simulink model "spiBitbangSimulink_So2"  (R2013b)
settings: Solver=FixedStepDiscrete  SolverMode=SingleTasking  StartTime=0.0  StopTime=4e-3  FixedStep=sampleTime  MaxStep=MaxStepSize  RelTol=1e-3
undefined symbols (not defined in the file or in its folder): Low, periSam, sampleTime, sampleTIme, sigbuilder_block
libraries: simulink_extras x30, simulink x16, dspswit3 x8, embdlinuxlib x5, powerlib_meascontrol x2, dspsnks4 x1
settings Model: ExtModeTrigDuration=100  Creator=mainster  LastModifiedBy=mainster
settings OptimizationCC: OptimizeModelRefInitCode=on  LifeSpan=1
settings DebuggingCC: SolverPrmCheckMsg=none  InheritedTsInSrcMsg=none
settings HardwareCC: ProdLargestAtomicInteger=Long  ProdLargestAtomicFloat=Double  ProdEndianess=LittleEndian  ProdHWDeviceType=ARM Compatible->ARM Cortex
settings RTWCC: SystemTargetFile=realtime.tlc  GenerateMakefile=off  TemplateMakefile=realtime.tmf  Description=Run on Target Hardware  RTWVerbose=off  ProcessScript=realtime_make_rtw_hook
settings STFCustomTargetCC: TargetLibSuffix=.a  GenerateSampleERTMain=on  ERTCustomFileBanners=on  SupportNonInlinedSFcns=off  SupportVariableSizeSignals=on  MATLABClassNameForMDSCustomization=Simulink.SoftwareTarget.ERTCustomization  GRTInterface=off  SystemTargetFile=realtime.tlc
settings ERTTargetCC: CodeReplacementLibrary=ANSI_C  GenerateSampleERTMain=on  ParMdlRefBuildCompliant=off  CompOptLevelCompliant=off  ConcurrentExecutionCompliant=off  CombineOutputUpdateFcns=off  ERTFirstTimeCompliant=off  SupportContinuousTime=on  SupportVariableSizeSignals=on  ModelStepFunctionPrototypeControlCompliant=off  CPPClassGenCompliant=off  ExtModeMexArgs='192.168.2.111' 0 17725  InlinedParameterPlacement=NonHierarchical  ERTSrcFileBannerTemplate=realtime_code_template.cgt  ERTHdrFileBannerTemplate=realtime_code_template.cgt  ERTDataSrcFileTemplate=realtime_code_template.cgt  ERTDataHdrFileTemplate=realtime_code_template.cgt  ERTCustomFileTemplate=realtime_file_process.tlc
settings ConfigurationSet: Description=SimMechanics 2G

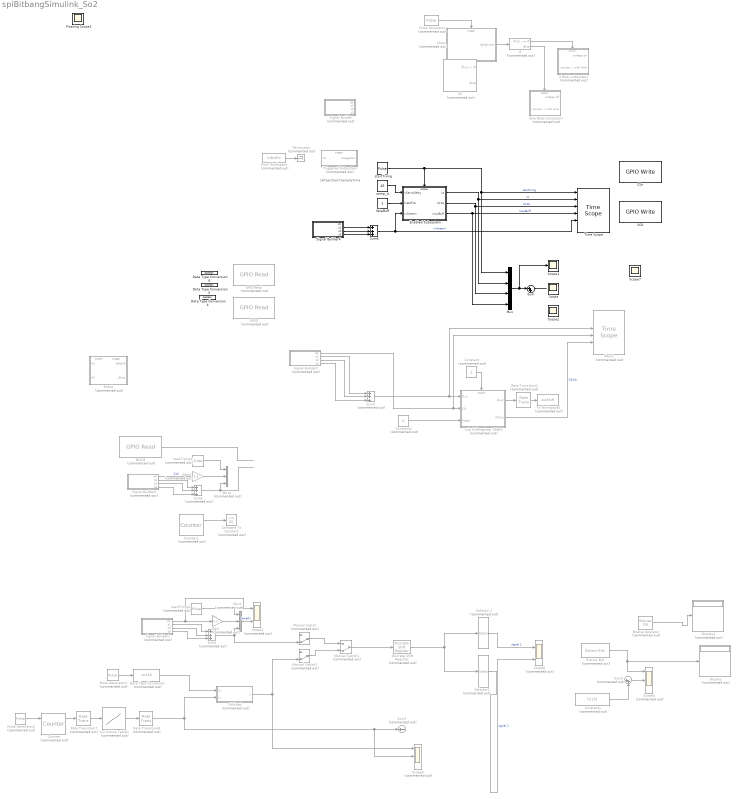
== system spiBitbangSimulink_So2 ==
  note: 16*periSam*sampleTime
  " ShiftLeft" : Subsystem  Commented=on  TreatAsAtomicUnit=on
  1-D Lookup Table1 : Lookup_n-D  Commented=on  NumberOfTableDimensions=1  BreakpointsForDimension1=[0,1,2,3,4]  IndexSearchMethod=Evenly spaced points  UseOneInputPortForAllInputData=on  Table=[3325,6553,44558,8856,60254]  TableDataTypeStr=uint16  InterpMethod=Flat  SampleTime=sampleTime  InternalRulePriority=Speed  OutDataTypeStr=uint16  RndMeth=Simplest  InputSameDT=on
  Bitwise Operator : simulink/Logic and Bit Operations/Bitwise Operator  Commented=on  logicop=OR  UseBitMask=off  BitMask=bin2dec('11011001')  BitMaskRealWorld=Real World Value
  CSn : embdlinuxlib/GPIO Write  board=Model B Rev2  gpio=27  direction=Output  blockPlatform=Raspberry Pi
  Chart : Stateflow chart  Commented=on  TreatAsAtomicUnit=on
  Compare To Constant : simulink/Logic and Bit Operations/Compare To Constant  Commented=on  relop=<=  const=25  OutDataTypeStr=boolean  ZeroCross=off
  Constant : Constant  Commented=on  SampleTime=-1
  Constant1 : Constant  Commented=on  Value=[0:15]  VectorParams1D=off  SampleTime=sampleTIme
      settings: SamplingMode=Frame based
  Constant2 : Constant  Commented=on  Value=0  OutDataTypeStr=Inherit: Inherit via back propagation  SampleTime=-1
  Counter : dspswit3/Counter  Commented=on  Direction=Up  CountEvent=Rising edge  CounterSize=User defined  MaxCount=5  InitialCount=1  Output=Count and Hit  HitValue=32  ResetInput=on  SamplesPerFrame=1  Ts=1  CntDtype=double  HitDtype=Logical
  Counter1 : dspswit3/Counter  Commented=on  Direction=Up  CountEvent=Rising edge  CounterSize=User defined  MaxCount=255  InitialCount=0  Output=Count and Hit  HitValue=32  ResetInput=on  SamplesPerFrame=1  Ts=1  CntDtype=double  HitDtype=Boolean
  Data Type Conversion : DataTypeConversion  Commented=on  OutDataTypeStr=uint16
  Data Type Conversion4 : DataTypeConversion  OutDataTypeStr=boolean
  Data Type Conversion5 : DataTypeConversion  OutDataTypeStr=boolean
  Data Type Conversion6 : DataTypeConversion  OutDataTypeStr=boolean
  Discrete Shift Register : powerlib_meascontrol/Additional Components/Discrete Shift Register  Commented=on  NSamples=16  InitialValue=0  Ts=periSam*sampleTime
  Display : Display  Commented=on
      settings: Format=decimal (Stored Integer)
  Display1 : Display  Commented=on
      settings: Format=decimal (Stored Integer)
  Else Body subsystem : Subsystem  Commented=on  TreatAsAtomicUnit=on
  Enabled Subsystem : Subsystem  TreatAsAtomicUnit=on
  Extract Bits : simulink/Logic and Bit Operations/Extract Bits  Commented=on  bitsToExtract=Range of bits  numBits=8  bitIdxRange=[0 0]  outScalingMode=Treat bit field as an integer
  From Workspace : FromWorkspace  Commented=on  VariableName=txBuffIn  SampleTime=0
  GPIO Read : embdlinuxlib/GPIO Read  Commented=on  board=Model B Rev2  gpio=4  internalResistor=Off  sampleTime=0.1  direction=Input  blockPlatform=Raspberry Pi
  Gain : Gain  Commented=on  Gain=1.1  SampleTime=sampleTime
  Gain2 : Gain  Commented=on  Gain=1.1  SampleTime=sampleTime
  If : If  Commented=on  IfExpression=u1 ~= 0
  If Body subsystem : Subsystem  Commented=on  TreatAsAtomicUnit=on
  If1 : If  Commented=on  NumInputs=2
  MISO : embdlinuxlib/GPIO Read  Commented=on  board=Model B Rev2  gpio=24  internalResistor=Off  sampleTime=0.1  direction=Input  blockPlatform=Raspberry Pi
  MISO1 : embdlinuxlib/GPIO Read  Commented=on  board=Model B Rev2  gpio=4  internalResistor=Off  sampleTime=0.1  direction=Input  blockPlatform=Raspberry Pi
  Main1 : TimeScope  Commented=on  NumInputPorts=6  DefaultConfigurationName=spbscopes.TimeScopeBlockCfg
      settings: CopyFcn=scopeextensions.ScopeBlock.onCoreBlockCopy(gcbh);  DeleteFcn=scopeextensions.ScopeBlock.callback(gcbh, 'onBlockDelete');  PreSaveFcn=scopeextensions.ScopeBlock.callback(gcbh, 'onModelSave');  NameChangeFcn=scopeextensions.ScopeBlock.callback(gcbh, 'onBlockRename');  DestroyFcn=scopeextensions.ScopeBlock.onBlockDestroy(gcbh)  CloseFcn=scopeextensions.ScopeBlock.callback(gcbh, 'onBlockClose');  PreDeleteFcn=scopeextensions.ScopeBlock.callback(gcbh, 'onBlockPreDelete');
  Manual Switch : ManualSwitch  Commented=on  CurrentSetting=0
  Manual Switch1 : ManualSwitch  Commented=on  CurrentSetting=0
  Manual Switch2 : ManualSwitch  Commented=on  CurrentSetting=0
  Mux : Mux
  Mux1 : Mux  Commented=on  Inputs=3
  Mux4 : Mux  Commented=on  Inputs=3
  Pulse Generator : DiscretePulseGenerator  Commented=on  Period=periSam  PulseWidth=periSam/2  SampleTime=-1
  Pulse Generator1 : DiscretePulseGenerator  Commented=on  Period=periSam  PulseWidth=periSam/2  SampleTime=periSam*sampleTime
  Pulse Generator2 : DiscretePulseGenerator  Commented=on  Period=periSam*16  PulseWidth=8*periSam  SampleTime=sampleTime
  Rate Transition1 : RateTransition  Commented=on  OutPortSampleTime=sampleTime*periSam
  Rate Transition7 : RateTransition  Commented=on  OutPortSampleTime=sampleTime
  Rate Transition8 : RateTransition  Commented=on  OutPortSampleTime=periSam*sampleTime
  RxSub : Subsystem  Commented=on  TreatAsAtomicUnit=on
  SCK : embdlinuxlib/GPIO Write  board=Model B Rev2  gpio=17  direction=Output  blockPlatform=Raspberry Pi
  Scope : Scope
      settings: Floating=on  ShowLegends=on  TimeRange=0.002  YMin=-0.2
  Scope1 : Scope
      settings: ShowLegends=on  TimeRange=0.002  YMin=-0.2
  Scope2 : Scope  NumInputPorts=4
      settings: Floating=on  ShowLegends=on  TimeRange=0.002  YMin=-0.2~-0.2~-0.2~-0.2  YMax=1.2~1.2~1.2~18  SaveName=ScopeData2
  Scope3 : Scope  Commented=on  NumInputPorts=2
      settings: ShowLegends=on  TimeRange=0.00032  YMin=-0.2~-5  YMax=1.6~5  SaveName=ScopeData4  SampleInput=on
  Scope4 : Scope  Commented=on  NumInputPorts=3
      settings: ShowLegends=on  TimeRange=0.00032  YMin=-0.2~-5~-5  YMax=1.6~5~5  SaveName=ScopeData5  SampleInput=on
  Scope5 : Scope  Commented=on  NumInputPorts=3
      settings: ShowLegends=on  TimeRange=0.00032  YMin=-0.2~-5~-5  YMax=1.6~5~5  SaveName=ScopeData6  SampleInput=on
  Scope6 : Scope  Commented=on  NumInputPorts=2
      settings: TimeRange=0.03  YMin=-1~-1  YMax=1~1  SaveName=ScopeData7
  Scope7 : Scope  NumInputPorts=4
      settings: ShowLegends=on  TimeRange=0.004  YMin=-0.2~-0.2~-0.2~-0.2  YMax=1.2~1.2~1.2~18  SaveName=ScopeData9
  Selector 1 : Selector  Commented=on  InputPortWidth=16  IndexOptions=Index vector (dialog)  Indices=[1:8]  OutputSizes=1
  Selector2 : Selector  Commented=on  InputPortWidth=16  IndexOptions=Index vector (dialog)  Indices=[9:16]  OutputSizes=1
  Signal Builder : Subsystem  Tag=STV Subsys  Commented=on  LoadFcn=sigbuilder_block('load');  StartFcn=sigbuilder_block('start');  StopFcn=sigbuilder_block('stop');  ClipboardFcn=sigbuilder_block('clipboard');  mask(Sigbuilder block){}
      mask help: Simulink:masks:SigbuilderBlock_MD
      mask init:
      | if ~strcmp(get_param(bdroot(gcbh),'SimulationStatus'),'stopped') tuvar = sigbuilder_block('maskInit'); end
      settings: CopyFcn=sigbuilder_block('copy');  DeleteFcn=sigbuilder_block('delete');  ModelCloseFcn=sigbuilder_block('modelClose');  PreSaveFcn=sigbuilder_block('preSave');  PauseFcn=sigbuilder_block('pause');  ContinueFcn=sigbuilder_block('continue');  NameChangeFcn=sigbuilder_block('namechange');  OpenFcn=sigbuilder_block('open',[141 95.25 837.75 399.75 ]);  CloseFcn=sigbuilder_block('close');
      mask Display: plot(0, 0, 100, 100,[2, 2, 32, 32, 2], [68, 8, 8, 68, 68],[32, 2], [38, 38], [32, 19, 2],[53, 60, 44], [32, 17, 17, 2],[16, 16, 31, 31]);txt = getActiveGroup(gcbh);text(2, 100, txt,'verticalAlignment', 'top');
  Signal Builder1 : Subsystem  Tag=STV Subsys  Commented=on  LoadFcn=sigbuilder_block('load');  StartFcn=sigbuilder_block('start');  StopFcn=sigbuilder_block('stop');  ClipboardFcn=sigbuilder_block('clipboard');  mask(Sigbuilder block){}
      mask help: Simulink:masks:SigbuilderBlock_MD
      mask init:
      | if ~strcmp(get_param(bdroot(gcbh),'SimulationStatus'),'stopped') tuvar = sigbuilder_block('maskInit'); end
      settings: CopyFcn=sigbuilder_block('copy');  DeleteFcn=sigbuilder_block('delete');  ModelCloseFcn=sigbuilder_block('modelClose');  PreSaveFcn=sigbuilder_block('preSave');  PauseFcn=sigbuilder_block('pause');  ContinueFcn=sigbuilder_block('continue');  NameChangeFcn=sigbuilder_block('namechange');  OpenFcn=sigbuilder_block('open',[367.5 138 550.5 399.75 ]);  CloseFcn=sigbuilder_block('close');
      mask Display: plot(0, 0, 100, 100,[2, 2, 32, 32, 2], [68, 8, 8, 68, 68],[32, 2], [38, 38], [32, 19, 2],[53, 60, 44], [32, 17, 17, 2],[16, 16, 31, 31]);txt = getActiveGroup(gcbh);text(2, 100, txt,'verticalAlignment', 'top');
  Signal Builder2 : Subsystem  Tag=STV Subsys  Commented=on  LoadFcn=sigbuilder_block('load');  StartFcn=sigbuilder_block('start');  StopFcn=sigbuilder_block('stop');  ClipboardFcn=sigbuilder_block('clipboard');  TreatAsAtomicUnit=on  mask(Sigbuilder block){}
      mask help: Simulink:masks:SigbuilderBlock_MD
      mask init:
      | if ~strcmp(get_param(bdroot(gcbh),'SimulationStatus'),'stopped') tuvar = sigbuilder_block('maskInit'); end
      settings: CopyFcn=sigbuilder_block('copy');  DeleteFcn=sigbuilder_block('delete');  ModelCloseFcn=sigbuilder_block('modelClose');  PreSaveFcn=sigbuilder_block('preSave');  PauseFcn=sigbuilder_block('pause');  ContinueFcn=sigbuilder_block('continue');  NameChangeFcn=sigbuilder_block('namechange');  OpenFcn=sigbuilder_block('open',[367.5 138 550.5 399.75 ]);  CloseFcn=sigbuilder_block('close');
      mask Display: plot(0, 0, 100, 100,[2, 2, 32, 32, 2], [68, 8, 8, 68, 68],[32, 2], [38, 38], [32, 19, 2],[53, 60, 44], [32, 17, 17, 2],[16, 16, 31, 31]);txt = getActiveGroup(gcbh);text(2, 100, txt,'verticalAlignment', 'top');
  Signal Builder3 : Subsystem  Tag=STV Subsys  Commented=on  LoadFcn=sigbuilder_block('load');  StartFcn=sigbuilder_block('start');  StopFcn=sigbuilder_block('stop');  ClipboardFcn=sigbuilder_block('clipboard');  SystemSampleTime=sampleTime  mask(Sigbuilder block){}
      mask help: Simulink:masks:SigbuilderBlock_MD
      mask init:
      | if ~strcmp(get_param(bdroot(gcbh),'SimulationStatus'),'stopped') tuvar = sigbuilder_block('maskInit'); end
      settings: CopyFcn=sigbuilder_block('copy');  DeleteFcn=sigbuilder_block('delete');  ModelCloseFcn=sigbuilder_block('modelClose');  PreSaveFcn=sigbuilder_block('preSave');  PauseFcn=sigbuilder_block('pause');  ContinueFcn=sigbuilder_block('continue');  NameChangeFcn=sigbuilder_block('namechange');  OpenFcn=sigbuilder_block('open',[367.5 138 550.5 399.75 ]);  CloseFcn=sigbuilder_block('close');
      mask Display: plot(0, 0, 100, 100,[2, 2, 32, 32, 2], [68, 8, 8, 68, 68],[32, 2], [38, 38], [32, 19, 2],[53, 60, 44], [32, 17, 17, 2],[16, 16, 31, 31]);txt = getActiveGroup(gcbh);text(2, 100, txt,'verticalAlignment', 'top');
  Signal Builder4 : Subsystem  Tag=STV Subsys  LoadFcn=sigbuilder_block('load');  StartFcn=sigbuilder_block('start');  StopFcn=sigbuilder_block('stop');  ClipboardFcn=sigbuilder_block('clipboard');  TreatAsAtomicUnit=on  mask(Sigbuilder block){}
      mask help: Simulink:masks:SigbuilderBlock_MD
      mask init:
      | if ~strcmp(get_param(bdroot(gcbh),'SimulationStatus'),'stopped') tuvar = sigbuilder_block('maskInit'); end
      settings: CopyFcn=sigbuilder_block('copy');  DeleteFcn=sigbuilder_block('delete');  ModelCloseFcn=sigbuilder_block('modelClose');  PreSaveFcn=sigbuilder_block('preSave');  PauseFcn=sigbuilder_block('pause');  ContinueFcn=sigbuilder_block('continue');  NameChangeFcn=sigbuilder_block('namechange');  OpenFcn=sigbuilder_block('open',[367.5 138 550.5 399.75 ]);  CloseFcn=sigbuilder_block('close');
      mask Display: plot(0, 0, 100, 100,[2, 2, 32, 32, 2], [68, 8, 8, 68, 68],[32, 2], [38, 38], [32, 19, 2],[53, 60, 44], [32, 17, 17, 2],[16, 16, 31, 31]);txt = getActiveGroup(gcbh);text(2, 100, txt,'verticalAlignment', 'top');
  Sum : Sum  Inputs=|++  LockScale=on
  Sum1 : Sum  Commented=on  Inputs=+++  SampleTime=sampleTime
  Sum2 : Sum  Commented=on  Inputs=|++  LockScale=on
  Sum3 : Sum  Commented=on  Inputs=+-
  Sum4 : Sum  Commented=on  Inputs=+++  SampleTime=sampleTime
  Sum5 : Sum  Commented=on  Inputs=+++  SampleTime=sampleTime
  Sum6 : Sum  Inputs=+++  SampleTime=sampleTime
  Terminator : Terminator  Commented=on
  Time Scope : TimeScope  NumInputPorts=6  DefaultConfigurationName=spbscopes.TimeScopeBlockCfg
      settings: CopyFcn=scopeextensions.ScopeBlock.onCoreBlockCopy(gcbh);  DeleteFcn=scopeextensions.ScopeBlock.callback(gcbh, 'onBlockDelete');  PreSaveFcn=scopeextensions.ScopeBlock.callback(gcbh, 'onModelSave');  NameChangeFcn=scopeextensions.ScopeBlock.callback(gcbh, 'onBlockRename');  DestroyFcn=scopeextensions.ScopeBlock.onBlockDestroy(gcbh)  CloseFcn=scopeextensions.ScopeBlock.callback(gcbh, 'onBlockClose');  PreDeleteFcn=scopeextensions.ScopeBlock.callback(gcbh, 'onBlockPreDelete');
  To Workspace1 : ToWorkspace  Commented=on  VariableName=outShift  SampleTime=periSam*sampleTime  SaveFormat=Timeseries
  Triggered Subsystem : Subsystem  Commented=on  TreatAsAtomicUnit=on
  fakeBuff : Constant
  samp_tL : Constant  Value=25
  startTixing : DiscretePulseGenerator  Period=800  PulseWidth=700  SampleTime=sampleTime
  startTixing1 : DiscretePulseGenerator  Commented=on  Period=periSam  PulseWidth=periSam*0.1  SampleTime=sampleTime
  startTixing2 : DiscretePulseGenerator  Commented=on  Period=periSam  PulseWidth=periSam*0.1  SampleTime=sampleTime
  sub Shiftregister 16Bit1 : Subsystem  Commented=on  TreatAsAtomicUnit=on
  Floating Scope1 : Scope
      settings: Floating=on  SaveName=ScopeData3
  wires:
  startTixing/1 -> Enabled Subsystem/Enable, Mux/1, Time Scope/1  "startTxing"
  Pulse Generator/1 -> Chart/Trigger
  Chart/1(lightSwitch) -> If/1
  If/1 -> If Body subsystem/Action
  If/2 -> Else Body subsystem/Action
  Enabled Subsystem/2(clk16) -> Mux/3, Time Scope/3  "clk16"
  Enabled Subsystem/1(cs) -> Mux/2, Time Scope/2  "cs"
  Sum/1 -> ?
  samp_tL/1 -> Enabled Subsystem/1(nSampDelay)
  fakeBuff/1 -> Enabled Subsystem/2(txBuff16)
  Enabled Subsystem/3(mosiBuff) -> Mux/4, Time Scope/4  "mosiBuff"
  From Workspace/1 -> Terminator/1
  Mux/1 -> Scope1/1, Sum/1
  Signal Builder1/3(s2) -> Sum1/2
  Signal Builder1/2(s1) -> Sum1/1
  Signal Builder1/4(s3) -> Sum1/3
  Sum1/1 -> Manual Switch/2, Mux1/3
  startTixing1/1 -> Mux1/1
  Gain/1 -> Mux1/2
  Manual Switch1/1 -> Discrete Shift Register/1
  Mux1/1 -> Scope3/2  "fakeRx"
  Signal Builder1/1(clk) -> Scope3/1, Gain/1
  Manual Switch/1 -> Manual Switch1/1
  Manual Switch2/1 -> Manual Switch1/2
  " ShiftLeft"/1(y) -> Scope5/1, Manual Switch2/2
  Constant1/1 -> Sum2/2
  Sum2/1 -> Scope4/2
  Pulse Generator1/1 -> Data Type Conversion/1
  Rate Transition8/1 -> " ShiftLeft"/2(in), Scope5/2, Sum3/1
  Rate Transition7/1 -> 1-D Lookup Table1/1
  1-D Lookup Table1/1 -> Rate Transition8/1
  Pulse Generator2/1 -> Counter/1
  Counter/1 -> Rate Transition7/1
  Data Type Conversion/1 -> " ShiftLeft"/1(ld)
  Extract Bits/1 -> Display/1, Scope4/1
  ? -> Bitwise Operator/1
  Bitwise Operator/1 -> Display1/1
  Selector 1/1 -> Scope6/1  "signal 1"
  Selector2/1 -> Scope6/2  "signal 2"
  Discrete Shift Register/1 -> Selector 1/1, Selector2/1
  Signal Builder3/3(s2) -> Sum5/2
  Signal Builder3/2(s1) -> Sum5/1
  Signal Builder3/4(s3) -> Sum5/3
  Sum5/1 -> Mux4/3
  startTixing2/1 -> Mux4/1
  Gain2/1 -> Mux4/2
  Signal Builder3/1(clk) -> Gain2/1  "CLK"
  MISO1/1 -> ?
  Counter1/1 -> Compare To Constant/1
  Signal Builder2/3(s2) -> Sum4/2
  Signal Builder2/2(s1) -> Sum4/1
  Signal Builder2/4(s3) -> Sum4/3
  Rate Transition1/1 -> To Workspace1/1
  sub Shiftregister 16Bit1/1(Dout) -> Rate Transition1/1
  Constant2/1 -> sub Shiftregister 16Bit1/3(Reset)
  Signal Builder2/1(clk) -> Main1/4, sub Shiftregister 16Bit1/2(Clk)
  Sum4/1 -> Main1/3, sub Shiftregister 16Bit1/1(D_in)
  sub Shiftregister 16Bit1/2(ClkCtr) -> Main1/5  "ClkCtr"
  Constant/1 -> sub Shiftregister 16Bit1/Enable
  Signal Builder4/3(s2) -> Sum6/2
  Signal Builder4/2(s1) -> Sum6/1
  Signal Builder4/4(s3) -> Sum6/3
  Sum6/1 -> Enabled Subsystem/3(rxStream), Time Scope/5  "rxStream"

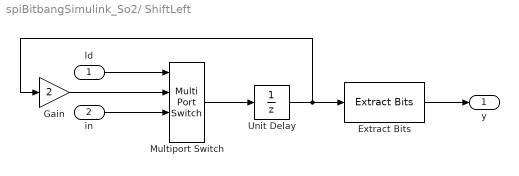
== system spiBitbangSimulink_So2/ ShiftLeft ==
  ld : Inport  OutDataTypeStr=uint16
  in : Inport  Port=2
  Extract Bits : simulink/Logic and Bit Operations/Extract Bits  bitsToExtract=Lower half  numBits=8  bitIdxRange=[0 15]  outScalingMode=Treat bit field as an integer
  Gain : Gain  Gain=2  ParamDataTypeStr=Inherit: Inherit from 'Gain'  OutDataTypeStr=Inherit: Inherit via back propagation
  Multiport Switch : MultiPortSwitch  DataPortOrder=Zero-based contiguous  DiagnosticForDefault=Warning
  Unit Delay : UnitDelay  SampleTime=-1
  y : Outport  PortDimensions=1
  wires:
  ld/1 -> Multiport Switch/1
  in/1 -> Multiport Switch/3
  Gain/1 -> Multiport Switch/2
  Multiport Switch/1 -> Unit Delay/1
  Unit Delay/1 -> Gain/1, Extract Bits/1
  Extract Bits/1 -> y/1

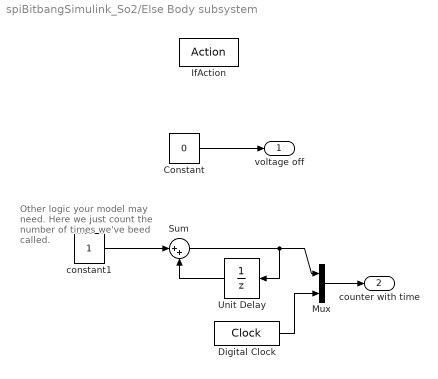
== system spiBitbangSimulink_So2/Else Body subsystem ==
  note: Other logic your model may need. Here we just count the number
      | of times we've beed called.
  IfAction : ActionPort
  Constant : Constant  Value=0
  Digital Clock : DigitalClock
  Mux : Mux  Inputs=2
  Sum : Sum  Inputs=|++  SaturateOnIntegerOverflow=on  InputSameDT=on  OutDataTypeStr=Inherit: Same as first input
  Unit Delay : UnitDelay
  constant1 : Constant
  voltage off : Outport  InitialOutput=0
  counter with time : Outport  Port=2
  wires:
  Constant/1 -> voltage off/1
  Sum/1 -> Mux/1, Unit Delay/1
  constant1/1 -> Sum/1
  Unit Delay/1 -> Sum/2
  Mux/1 -> counter with time/1
  Digital Clock/1 -> Mux/2

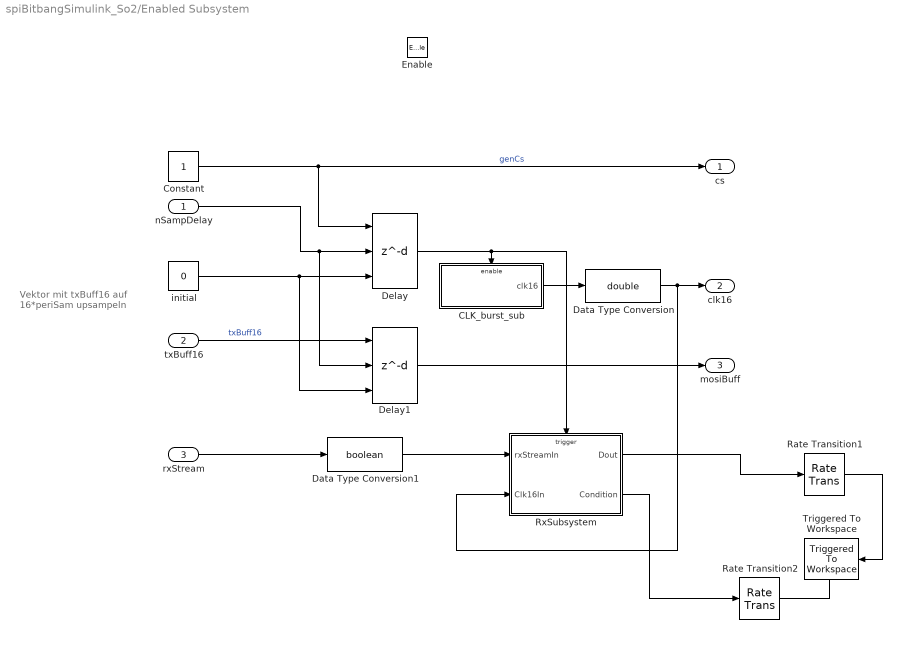
== system spiBitbangSimulink_So2/Enabled Subsystem ==
  note: Vektor mit txBuff16 auf
      | 16*periSam upsampeln
  nSampDelay : Inport
  txBuff16 : Inport  Port=2
  rxStream : Inport  Port=3
  Enable : EnablePort  StatesWhenEnabling=reset
  CLK_burst_sub : Subsystem  TreatAsAtomicUnit=on
  Constant : Constant
  Data Type Conversion : DataTypeConversion  OutDataTypeStr=double
  Data Type Conversion1 : DataTypeConversion  OutDataTypeStr=boolean
  Delay : Delay  DelayLengthSource=Input port  DelayLength=1  InitialConditionSource=Input port  InitialCondition=0  InputProcessing=Inherited
      settings: InputPortMap=u0,p1,p4
  Delay1 : Delay  DelayLengthSource=Input port  DelayLength=1  InitialConditionSource=Input port  InitialCondition=0  InputProcessing=Inherited
      settings: InputPortMap=u0,p1,p4
  Rate Transition1 : RateTransition  OutPortSampleTime=sampleTime*periSam
  Rate Transition2 : RateTransition  OutPortSampleTime=sampleTime*periSam
  RxSubsystem : Subsystem  TreatAsAtomicUnit=on
  "Triggered To Workspace\t" : dspsnks4/Triggered To Workspace  TriggerType=Falling edge  VariableName=youtFull  Buffer=10  Save2DMode=2-D array (concatenate along first dimension)
      settings: FixptAsFi=off
  initial : Constant  Value=0
  cs : Outport  InitialOutput=1
  clk16 : Outport  Port=2  InitialOutput=0
  mosiBuff : Outport  Port=3  InitialOutput=0
  wires:
  CLK_burst_sub/1(clk16) -> Data Type Conversion/1
  nSampDelay/1 -> Delay1/2, Delay/2
  initial/1 -> Delay1/3, Delay/3
  Constant/1 -> cs/1, Delay/1  "genCs"
  Delay/1 -> RxSubsystem/Trigger, CLK_burst_sub/Enable
  txBuff16/1 -> Delay1/1  "txBuff16"
  Delay1/1 -> mosiBuff/1
  Data Type Conversion/1 -> RxSubsystem/2(Clk16In), clk16/1
  rxStream/1 -> Data Type Conversion1/1
  Data Type Conversion1/1 -> RxSubsystem/1(rxStreamIn)
  Rate Transition1/1 -> "Triggered To Workspace\t"/1
  Rate Transition2/1 -> "Triggered To Workspace\t"/Trigger
  RxSubsystem/1(Dout) -> Rate Transition1/1
  RxSubsystem/2(Condition) -> Rate Transition2/1

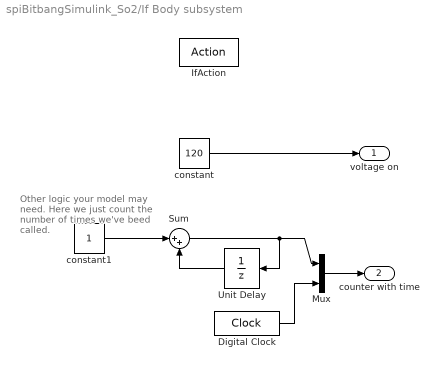
== system spiBitbangSimulink_So2/If Body subsystem ==
  note: Other logic your model may need. Here we just count the number
      | of times we've beed called.
  IfAction : ActionPort
  Digital Clock : DigitalClock
  Mux : Mux  Inputs=2
  Sum : Sum  Inputs=|++  SaturateOnIntegerOverflow=on  InputSameDT=on  OutDataTypeStr=Inherit: Same as first input
  Unit Delay : UnitDelay
  constant : Constant  Value=120
  constant1 : Constant
  voltage on : Outport  InitialOutput=120
  counter with time : Outport  Port=2
  wires:
  constant/1 -> voltage on/1
  Sum/1 -> Unit Delay/1, Mux/1
  constant1/1 -> Sum/1
  Unit Delay/1 -> Sum/2
  Mux/1 -> counter with time/1
  Digital Clock/1 -> Mux/2

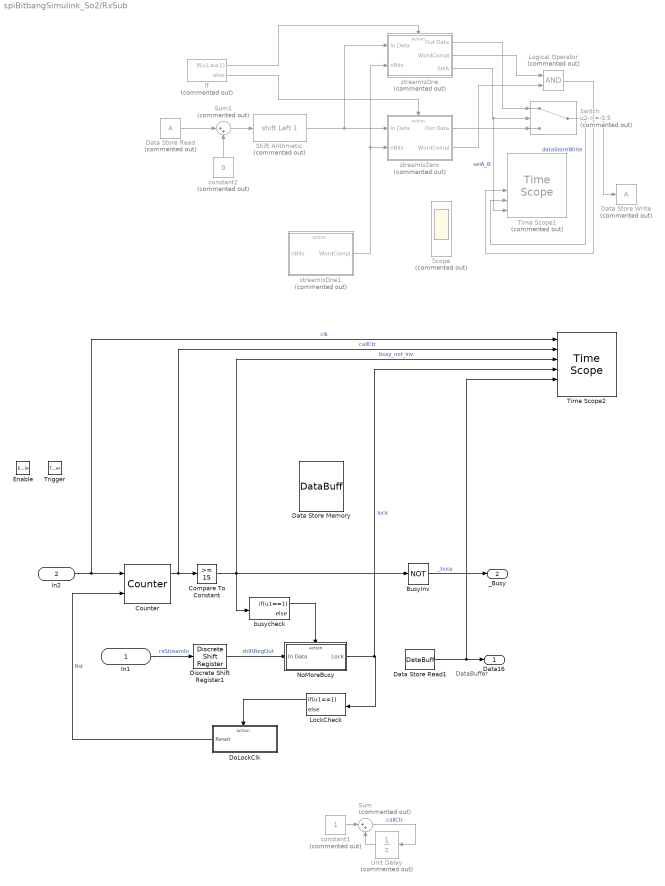
== system spiBitbangSimulink_So2/RxSub ==
  note: DataBuffer
  In1 : Inport
  In2 : Inport  Port=2
  Enable : EnablePort
  Trigger : TriggerPort  TriggerType=falling
  BusyInv : Logic  Operator=NOT  Inputs=1  IconShape=distinctive  AllPortsSameDT=off  OutDataTypeStr=boolean
  Compare To Constant : simulink/Logic and Bit Operations/Compare To Constant  relop=>=  const=15  OutDataTypeStr=boolean
  Counter : dspswit3/Counter  Direction=Up  CountEvent=Rising edge  CounterSize=User defined  MaxCount=255  InitialCount=0  Output=Count and Hit  HitValue=32  ResetInput=on  SamplesPerFrame=1  Ts=1  CntDtype=double  HitDtype=Logical
  Data Store Memory : DataStoreMemory  DataStoreName=DataBuff  ReadBeforeWriteMsg=warning  WriteAfterWriteMsg=warning  WriteAfterReadMsg=warning
  Data Store Read : DataStoreRead  Commented=on  DataStoreElements=A
  Data Store Read1 : DataStoreRead  DataStoreName=DataBuff  DataStoreElements=DataBuff
  Data Store Write : DataStoreWrite  Commented=on
  Discrete Shift Register1 : powerlib_meascontrol/Additional Components/Discrete Shift Register  NSamples=16  InitialValue=0  Ts=periSam*sampleTime
  DoLockClk : Subsystem  TreatAsAtomicUnit=on
  If : If  Commented=on  IfExpression=u1==1
  LockCheck : If  IfExpression=u1==1
  Logical Operator : Logic  Commented=on  AllPortsSameDT=off  OutDataTypeStr=boolean
  NoMoreBusy : Subsystem  TreatAsAtomicUnit=on
  Scope : Scope  Commented=on  NumInputPorts=6
      settings: ShowLegends=on  TimeRange=0.0045  YMin=-0.2~-5~-5~-5~-5~-5  YMax=5~5~5~5~5~5  SaveName=ScopeData8
  Shift Arithmetic : ArithShift  Commented=on  BitShiftNumber=1  BitShiftDirection=Left  DiagnosticForOORShift=Warning  CheckOORBitShift=on
  Sum : Sum  Commented=on  Inputs=|++  SaturateOnIntegerOverflow=on  InputSameDT=on  OutDataTypeStr=Inherit: Same as first input
  Sum1 : Sum  Commented=on  Inputs=|++  SaturateOnIntegerOverflow=on  InputSameDT=on  OutDataTypeStr=Inherit: Same as first input
  Switch : Switch  Commented=on  Threshold=0.5  OutDataTypeStr=uint16
  Time Scope1 : TimeScope  Commented=on  NumInputPorts=6  DefaultConfigurationName=spbscopes.TimeScopeBlockCfg
      settings: CopyFcn=scopeextensions.ScopeBlock.onCoreBlockCopy(gcbh);  DeleteFcn=scopeextensions.ScopeBlock.callback(gcbh, 'onBlockDelete');  PreSaveFcn=scopeextensions.ScopeBlock.callback(gcbh, 'onModelSave');  NameChangeFcn=scopeextensions.ScopeBlock.callback(gcbh, 'onBlockRename');  DestroyFcn=scopeextensions.ScopeBlock.onBlockDestroy(gcbh)  CloseFcn=scopeextensions.ScopeBlock.callback(gcbh, 'onBlockClose');  PreDeleteFcn=scopeextensions.ScopeBlock.callback(gcbh, 'onBlockPreDelete');
  Time Scope2 : TimeScope  NumInputPorts=6  DefaultConfigurationName=spbscopes.TimeScopeBlockCfg
      settings: CopyFcn=scopeextensions.ScopeBlock.onCoreBlockCopy(gcbh);  DeleteFcn=scopeextensions.ScopeBlock.callback(gcbh, 'onBlockDelete');  PreSaveFcn=scopeextensions.ScopeBlock.callback(gcbh, 'onModelSave');  NameChangeFcn=scopeextensions.ScopeBlock.callback(gcbh, 'onBlockRename');  DestroyFcn=scopeextensions.ScopeBlock.onBlockDestroy(gcbh)  CloseFcn=scopeextensions.ScopeBlock.callback(gcbh, 'onBlockClose');  PreDeleteFcn=scopeextensions.ScopeBlock.callback(gcbh, 'onBlockPreDelete');
  Unit Delay : UnitDelay  Commented=on  SampleTime=-1
  busycheck : If  IfExpression=u1==1
  constant1 : Constant  Commented=on  OutDataTypeStr=int8  SampleTime=-1  LockScale=on
  constant2 : Constant  Commented=on  Value=0  OutDataTypeStr=Inherit: Inherit via back propagation  SampleTime=-1  LockScale=on
  streamIsOne : Subsystem  Commented=on  TreatAsAtomicUnit=on
  streamIsOne1 : Subsystem  Commented=on  TreatAsAtomicUnit=on
  streamIsZero : Subsystem  Commented=on  TreatAsAtomicUnit=on
  Data16 : Outport
  _Busy : Outport  Port=2
  wires:
  If/2 -> streamIsZero/Action
  If/1 -> streamIsOne/Action
  Data Store Read/1 -> Sum1/1
  Sum1/1 -> Shift Arithmetic/1
  Shift Arithmetic/1 -> streamIsZero/1(In Data), streamIsOne/1(In Data)
  constant2/1 -> Sum1/2
  streamIsOne/3(SelA) -> Time Scope1/6, Switch/2  "selA_B"
  streamIsOne/1(Out Data) -> Switch/1
  streamIsZero/1(Out Data) -> Switch/3
  Switch/1 -> Time Scope1/5, Data Store Write/1  "dataStoreWrite"
  streamIsOne/2(WordCompl) -> Logical Operator/1
  streamIsZero/2(WordCompl) -> Logical Operator/2
  streamIsOne1/1(WordCompl) -> streamIsZero/2(nBits), streamIsOne/2(nBits)
  Logical Operator/1 -> Time Scope1/4
  Sum/1 -> Unit Delay/1  "callCtr"
  constant1/1 -> Sum/1
  Unit Delay/1 -> Sum/2
  In1/1 -> Discrete Shift Register1/1  "rxStreamIn"
  Compare To Constant/1 -> busycheck/1, Time Scope2/3, BusyInv/1  "busy_not_inv"
  Discrete Shift Register1/1 -> NoMoreBusy/1(In Data)  "shiftRegOut"
  BusyInv/1 -> _Busy/1  "_busy"
  busycheck/1 -> NoMoreBusy/Action
  Counter/1 -> Time Scope2/2, Compare To Constant/1  "callCtr"
  In2/1 -> Time Scope2/1, Counter/1  "clk"
  Data Store Read1/1 -> Time Scope2/5, Data16/1
  NoMoreBusy/1("Lock ") -> Time Scope2/4, LockCheck/1  "lock"
  LockCheck/1 -> DoLockClk/Action
  DoLockClk/1("Reset ") -> Counter/2  "Rst"

== system spiBitbangSimulink_So2/Signal Builder ==
  Demux : Demux  Tag=STV Demux
  FromWs : FromWorkspace  Tag=STV FromWs  VariableName=tuvar  SampleTime=100
      SigBuilderData=|
      | common.afterFinalStr = 'Extrapolate'
      | common.sampleTime = '100'
      | dataSet.timeRange = [0 32]
      | dataSet.name = 'Group 1'
      | sbobj.Groups.Name = 'Group 1'
      | sbobj.Groups.Signals(1).Name = 'clk'
      | sbobj.Groups.Signals(1).XData = [0 1 1 2 2 3 3 4 4 5 5 6 6 7 7 8 8 9 9 10 10 11 11 12 12 13 13 14 14 15 15 16 16 17 17 18 18 19 19 20 20 21 21 22 22 23 23 24 24 25 25 26 26 27 27 28 28 29 29 30 30 31 31 32]
      | sbobj.Groups.Signals(1).YData = [1 1 0 0 1 1 0 0 1 1 0 0 1 1 0 0 1 1 0 0 1 1 0 0 1 1 0 0 1 1 0 0 1 1 0 0 1 1 0 0 1 1 0 0 1 1 0 0 1 1 0 0 1 1 0 0 1 1 0 0 1 1 0 0]
      | sbobj.Groups.Signals(2).Name = 's1'
      | sbobj.Groups.Signals(2).XData = [0 0.5 0.5 1.52 1.52 32]
      | sbobj.Groups.Signals(2).YData = [0 0 1 1 0 0]
      | sbobj.Groups.Signals(3).Name = 's2'
      | sbobj.Groups.Signals(3).XData = [0 6 7.5 7.5 12.5 12.5 32]
      | sbobj.Groups.Signals(3).YData = [0 0 0 1 1 0 0]
      | sbobj.Groups.Signals(4).Name = 's3'
      | sbobj.Groups.Signals(4).XData = [0 17.5 17.5 29.5 29.5 32]
      | sbobj.Groups.Signals(4).YData = [0 0 1 1 0 0]
      | sbobj.Groups.TimeRange = [0 0.032]
  clk : Outport  Tag=STV Outport
  s1 : Outport  Tag=STV Outport  Port=2
  s2 : Outport  Tag=STV Outport  Port=3
  s3 : Outport  Tag=STV Outport  Port=4
  wires:
  FromWs/1 -> Demux/1
  Demux/1 -> clk/1
  Demux/2 -> s1/1
  Demux/3 -> s2/1
  Demux/4 -> s3/1

== system spiBitbangSimulink_So2/Signal Builder1 ==
  Demux : Demux  Tag=STV Demux
  FromWs : FromWorkspace  Tag=STV FromWs  VariableName=tuvar  SampleTime=0
      SigBuilderData=|
      | common.afterFinalStr = 'Extrapolate'
      | common.sampleTime = 0
      | dataSet.timeRange = [0 0.00032]
      | dataSet.name = 'Group 1'
      | sbobj.Groups.Name = 'Group 1'
      | sbobj.Groups.Signals(1).Name = 'clk'
      | sbobj.Groups.Signals(1).XData = [0 1e-05 1e-05 2e-05 2e-05 3e-05 3e-05 4e-05 4e-05 5e-05 5e-05 6e-05 6e-05 7e-05 7e-05 8e-05 8e-05 9e-05 9e-05 0.0001 0.0001 0.00011 0.00011 0.00012 0.00012 0.00013 0.00013 0.00014 0.00014 0.00015 0.00015 0.00016 0.00016 0.00017 0.00017 0.00018 0.00018 0.00019 0.00019 0.0002 0.0002 0.00021 0.00021 0.00022 0.00022 0.00023 0.00023 0.00024 0.00024 0.00025 0.00025 0.00026 0.00026 0.00027 0.00027 0.00028 0.00028 0.00029 0.00029 0.0003 0.0003 0.00031 0.00031 0.00032]
      | sbobj.Groups.Signals(1).YData = [1 1 0 0 1 1 0 0 1 1 0 0 1 1 0 0 1 1 0 0 1 1 0 0 1 1 0 0 1 1 0 0 1 1 0 0 1 1 0 0 1 1 0 0 1 1 0 0 1 1 0 0 1 1 0 0 1 1 0 0 1 1 0 0]
      | sbobj.Groups.Signals(2).Name = 's1'
      | sbobj.Groups.Signals(2).XData = [0 5e-06 5e-06 5.45e-05 5.45e-05 0.00032]
      | sbobj.Groups.Signals(2).YData = [0 0 1 1 0 0]
      | sbobj.Groups.Signals(3).Name = 's2'
      | sbobj.Groups.Signals(3).XData = [0 0.0001475 0.0001475 0.000196 0.000196 0.00032]
      | sbobj.Groups.Signals(3).YData = [0 0 1 1 0 0]
      | sbobj.Groups.Signals(4).Name = 's3'
      | sbobj.Groups.Signals(4).XData = [0 0.000237 0.000237 0.000297 0.000297 0.00032]
      | sbobj.Groups.Signals(4).YData = [0 0 1 1 0 0]
      | sbobj.Groups.TimeRange = [0 0.00032]
  clk : Outport  Tag=STV Outport
  s1 : Outport  Tag=STV Outport  Port=2
  s2 : Outport  Tag=STV Outport  Port=3
  s3 : Outport  Tag=STV Outport  Port=4
  wires:
  FromWs/1 -> Demux/1
  Demux/1 -> clk/1
  Demux/2 -> s1/1
  Demux/3 -> s2/1
  Demux/4 -> s3/1

== system spiBitbangSimulink_So2/Signal Builder2 ==
  Demux : Demux  Tag=STV Demux
  FromWs : FromWorkspace  Tag=STV FromWs  VariableName=tuvar  SampleTime=0
      SigBuilderData=|
      | common.afterFinalStr = 'Extrapolate'
      | common.sampleTime = 0
      | dataSet.timeRange = [0 0.00032]
      | dataSet.name = 'Group 1'
      | sbobj.Groups.Name = 'Group 1'
      | sbobj.Groups.Signals(1).Name = 'clk'
      | sbobj.Groups.Signals(1).XData = [0 1e-05 1e-05 2e-05 2e-05 3e-05 3e-05 4e-05 4e-05 5e-05 5e-05 6e-05 6e-05 7e-05 7e-05 8e-05 8e-05 9e-05 9e-05 0.0001 0.0001 0.00011 0.00011 0.00012 0.00012 0.00013 0.00013 0.00014 0.00014 0.00015 0.00015 0.00016 0.00016 0.00017 0.00017 0.00018 0.00018 0.00019 0.00019 0.0002 0.0002 0.00021 0.00021 0.00022 0.00022 0.00023 0.00023 0.00024 0.00024 0.00025 0.00025 0.00026 0.00026 0.00027 0.00027 0.00028 0.00028 0.00029 0.00029 0.0003 0.0003 0.00031 0.00031 0.00032]
      | sbobj.Groups.Signals(1).YData = [1 1 0 0 1 1 0 0 1 1 0 0 1 1 0 0 1 1 0 0 1 1 0 0 1 1 0 0 1 1 0 0 1 1 0 0 1 1 0 0 1 1 0 0 1 1 0 0 1 1 0 0 1 1 0 0 1 1 0 0 1 1 0 0]
      | sbobj.Groups.Signals(2).Name = 's1'
      | sbobj.Groups.Signals(2).XData = [0 5e-06 5e-06 5.45e-05 5.45e-05 0.00032]
      | sbobj.Groups.Signals(2).YData = [0 0 1 1 0 0]
      | sbobj.Groups.Signals(3).Name = 's2'
      | sbobj.Groups.Signals(3).XData = [0 0.0001475 0.0001475 0.000196 0.000196 0.00032]
      | sbobj.Groups.Signals(3).YData = [0 0 1 1 0 0]
      | sbobj.Groups.Signals(4).Name = 's3'
      | sbobj.Groups.Signals(4).XData = [0 0.000237 0.000237 0.000297 0.000297 0.00032]
      | sbobj.Groups.Signals(4).YData = [0 0 1 1 0 0]
      | sbobj.Groups.TimeRange = [0 0.00032]
  clk : Outport  Tag=STV Outport
  s1 : Outport  Tag=STV Outport  Port=2
  s2 : Outport  Tag=STV Outport  Port=3
  s3 : Outport  Tag=STV Outport  Port=4
  wires:
  FromWs/1 -> Demux/1
  Demux/1 -> clk/1
  Demux/2 -> s1/1
  Demux/3 -> s2/1
  Demux/4 -> s3/1

== system spiBitbangSimulink_So2/Signal Builder3 ==
  Demux : Demux  Tag=STV Demux
  FromWs : FromWorkspace  Tag=STV FromWs  VariableName=tuvar  SampleTime=0
      SigBuilderData=|
      | common.afterFinalStr = 'Extrapolate'
      | common.sampleTime = 0
      | dataSet.timeRange = [0 0.00032]
      | dataSet.name = 'Group 1'
      | sbobj.Groups.Name = 'Group 1'
      | sbobj.Groups.Signals(1).Name = 'clk'
      | sbobj.Groups.Signals(1).XData = [0 1e-05 1e-05 2e-05 2e-05 3e-05 3e-05 4e-05 4e-05 5e-05 5e-05 6e-05 6e-05 7e-05 7e-05 8e-05 8e-05 9e-05 9e-05 0.0001 0.0001 0.00011 0.00011 0.00012 0.00012 0.00013 0.00013 0.00014 0.00014 0.00015 0.00015 0.00016 0.00016 0.00017 0.00017 0.00018 0.00018 0.00019 0.00019 0.0002 0.0002 0.00021 0.00021 0.00022 0.00022 0.00023 0.00023 0.00024 0.00024 0.00025 0.00025 0.00026 0.00026 0.00027 0.00027 0.00028 0.00028 0.00029 0.00029 0.0003 0.0003 0.00031 0.00031 0.00032]
      | sbobj.Groups.Signals(1).YData = [1 1 0 0 1 1 0 0 1 1 0 0 1 1 0 0 1 1 0 0 1 1 0 0 1 1 0 0 1 1 0 0 1 1 0 0 1 1 0 0 1 1 0 0 1 1 0 0 1 1 0 0 1 1 0 0 1 1 0 0 1 1 0 0]
      | sbobj.Groups.Signals(2).Name = 's1'
      | sbobj.Groups.Signals(2).XData = [0 5e-06 5e-06 5.45e-05 5.45e-05 0.00032]
      | sbobj.Groups.Signals(2).YData = [0 0 1 1 0 0]
      | sbobj.Groups.Signals(3).Name = 's2'
      | sbobj.Groups.Signals(3).XData = [0 0.0001475 0.0001475 0.000196 0.000196 0.00032]
      | sbobj.Groups.Signals(3).YData = [0 0 1 1 0 0]
      | sbobj.Groups.Signals(4).Name = 's3'
      | sbobj.Groups.Signals(4).XData = [0 0.000237 0.000237 0.000297 0.000297 0.00032]
      | sbobj.Groups.Signals(4).YData = [0 0 1 1 0 0]
      | sbobj.Groups.TimeRange = [0 0.00032]
  clk : Outport  Tag=STV Outport
  s1 : Outport  Tag=STV Outport  Port=2
  s2 : Outport  Tag=STV Outport  Port=3
  s3 : Outport  Tag=STV Outport  Port=4
  wires:
  FromWs/1 -> Demux/1
  Demux/1 -> clk/1
  Demux/2 -> s1/1
  Demux/3 -> s2/1
  Demux/4 -> s3/1

== system spiBitbangSimulink_So2/Signal Builder4 ==
  Demux : Demux  Tag=STV Demux
  FromWs : FromWorkspace  Tag=STV FromWs  VariableName=tuvar  SampleTime=0
      SigBuilderData=|
      | common.afterFinalStr = 'Extrapolate'
      | common.sampleTime = 0
      | dataSet.timeRange = [0 0.00032]
      | dataSet.name = 'Group 1'
      | sbobj.Groups.Name = 'Group 1'
      | sbobj.Groups.Signals(1).Name = 'clk'
      | sbobj.Groups.Signals(1).XData = [0 1e-05 1e-05 2e-05 2e-05 3e-05 3e-05 4e-05 4e-05 5e-05 5e-05 6e-05 6e-05 7e-05 7e-05 8e-05 8e-05 9e-05 9e-05 0.0001 0.0001 0.00011 0.00011 0.00012 0.00012 0.00013 0.00013 0.00014 0.00014 0.00015 0.00015 0.00016 0.00016 0.00017 0.00017 0.00018 0.00018 0.00019 0.00019 0.0002 0.0002 0.00021 0.00021 0.00022 0.00022 0.00023 0.00023 0.00024 0.00024 0.00025 0.00025 0.00026 0.00026 0.00027 0.00027 0.00028 0.00028 0.00029 0.00029 0.0003 0.0003 0.00031 0.00031 0.00032]
      | sbobj.Groups.Signals(1).YData = [1 1 0 0 1 1 0 0 1 1 0 0 1 1 0 0 1 1 0 0 1 1 0 0 1 1 0 0 1 1 0 0 1 1 0 0 1 1 0 0 1 1 0 0 1 1 0 0 1 1 0 0 1 1 0 0 1 1 0 0 1 1 0 0]
      | sbobj.Groups.Signals(2).Name = 's1'
      | sbobj.Groups.Signals(2).XData = [0 5e-06 5e-06 5.45e-05 5.45e-05 0.00032]
      | sbobj.Groups.Signals(2).YData = [0 0 1 1 0 0]
      | sbobj.Groups.Signals(3).Name = 's2'
      | sbobj.Groups.Signals(3).XData = [0 0.0001475 0.0001475 0.000196 0.000196 0.00032]
      | sbobj.Groups.Signals(3).YData = [0 0 1 1 0 0]
      | sbobj.Groups.Signals(4).Name = 's3'
      | sbobj.Groups.Signals(4).XData = [0 0.000237 0.000237 0.000297 0.000297 0.00032]
      | sbobj.Groups.Signals(4).YData = [0 0 1 1 0 0]
      | sbobj.Groups.TimeRange = [0 0.00032]
  clk : Outport  Tag=STV Outport
  s1 : Outport  Tag=STV Outport  Port=2
  s2 : Outport  Tag=STV Outport  Port=3
  s3 : Outport  Tag=STV Outport  Port=4
  wires:
  FromWs/1 -> Demux/1
  Demux/1 -> clk/1
  Demux/2 -> s1/1
  Demux/3 -> s2/1
  Demux/4 -> s3/1

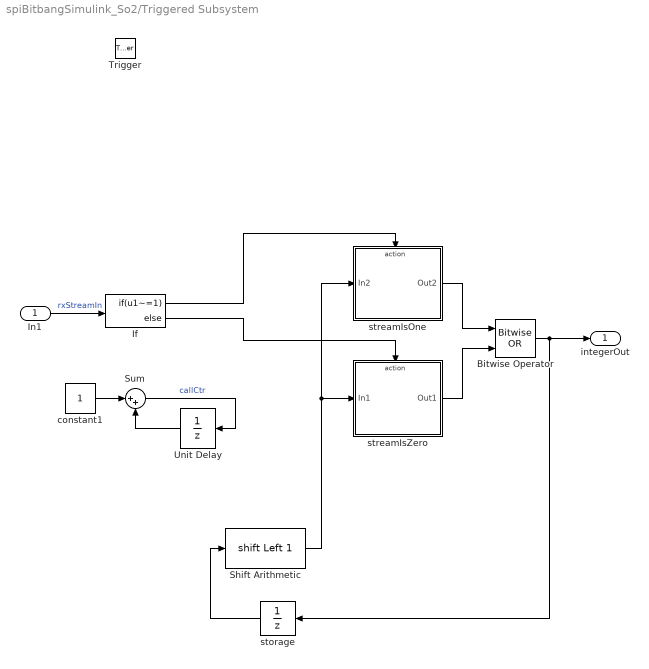
== system spiBitbangSimulink_So2/Triggered Subsystem ==
  In1 : Inport
  Trigger : TriggerPort  TriggerType=falling
  Bitwise Operator : simulink/Logic and Bit Operations/Bitwise Operator  logicop=OR  UseBitMask=off  NumInputPorts=2  BitMask=bin2dec('11011001')  BitMaskRealWorld=Stored Integer
  If : If  IfExpression=u1~=1
  Shift Arithmetic : ArithShift  BitShiftNumber=1  BitShiftDirection=Left  DiagnosticForOORShift=Warning  CheckOORBitShift=on
  Sum : Sum  Inputs=|++  SaturateOnIntegerOverflow=on  InputSameDT=on  OutDataTypeStr=Inherit: Same as first input
  Unit Delay : UnitDelay
  constant1 : Constant  OutDataTypeStr=int8  LockScale=on
  storage : UnitDelay  SampleTime=-1
  streamIsOne : Subsystem  TreatAsAtomicUnit=on
  streamIsZero : Subsystem  TreatAsAtomicUnit=on
  integerOut : Outport
  wires:
  In1/1 -> If/1  "rxStreamIn"
  Sum/1 -> Unit Delay/1  "callCtr"
  constant1/1 -> Sum/1
  Unit Delay/1 -> Sum/2
  Shift Arithmetic/1 -> streamIsOne/1(In2), streamIsZero/1(In1)
  storage/1 -> Shift Arithmetic/1
  If/2 -> streamIsZero/Action
  If/1 -> streamIsOne/Action
  streamIsOne/1(Out2) -> Bitwise Operator/1
  streamIsZero/1(Out1) -> Bitwise Operator/2
  Bitwise Operator/1 -> integerOut/1, storage/1

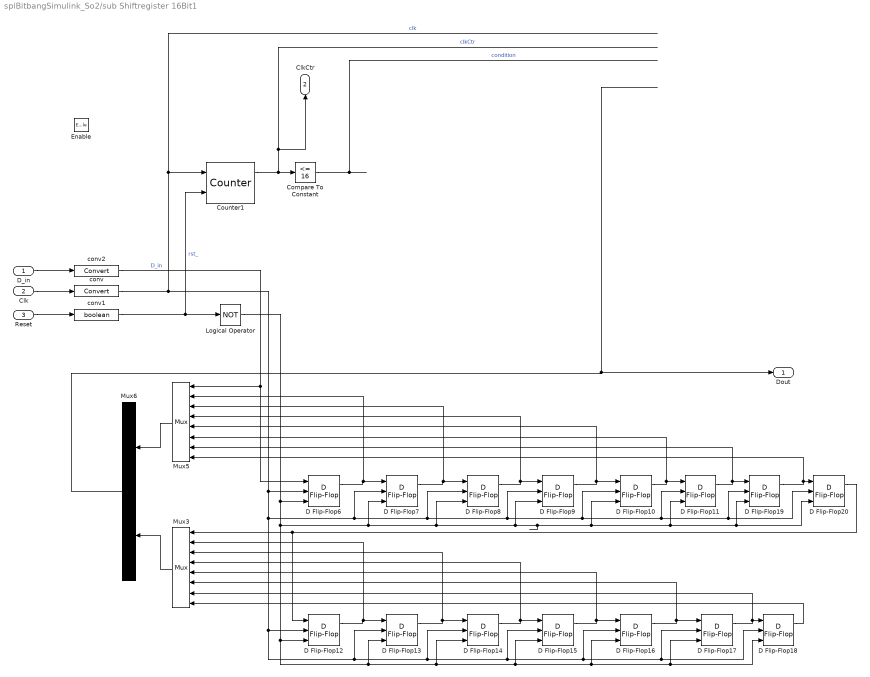
== system spiBitbangSimulink_So2/sub Shiftregister 16Bit1 ==
  D_in : Inport
  Clk : Inport  Port=2
  Reset : Inport  Port=3
  Enable : EnablePort  StatesWhenEnabling=reset
  Compare To Constant : simulink/Logic and Bit Operations/Compare To Constant  relop=<=  const=16  OutDataTypeStr=boolean  ZeroCross=off
  Counter1 : dspswit3/Counter  Direction=Up  CountEvent=Rising edge  CounterSize=User defined  MaxCount=255  InitialCount=0  Output=Count and Hit  HitValue=32  ResetInput=on  SamplesPerFrame=1  Ts=1  CntDtype=double  HitDtype=Boolean
  D Flip-Flop{6..20} (15 alike) : simulink_extras/Flip Flops/D Flip-Flop
  Logical Operator : Logic  Operator=NOT  IconShape=distinctive  AllPortsSameDT=off  OutDataTypeStr=boolean
  Mux3 : Mux  Inputs=8
  Mux5 : Mux  Inputs=8
  Mux6 : Mux  Inputs=2
  conv : DataTypeConversion  LockScale=on
  conv1 : DataTypeConversion  OutDataTypeStr=boolean
  conv2 : DataTypeConversion
  Dout : Outport
  ClkCtr : Outport  Port=2
  wires:
  D Flip-Flop6/1 -> Mux5/2, D Flip-Flop7/1
  D Flip-Flop7/1 -> Mux5/3, D Flip-Flop8/1
  D Flip-Flop9/1 -> Mux5/5, D Flip-Flop10/1
  D Flip-Flop10/1 -> Mux5/6, D Flip-Flop11/1
  D Flip-Flop12/1 -> Mux3/2, D Flip-Flop13/1
  D Flip-Flop13/1 -> Mux3/3, D Flip-Flop14/1
  D Flip-Flop14/1 -> Mux3/4, D Flip-Flop15/1
  D Flip-Flop17/1 -> Mux3/7, D Flip-Flop18/1
  conv/1 -> Counter1/1, D Flip-Flop13/2, D Flip-Flop16/2, D Flip-Flop17/2, D Flip-Flop18/2, D Flip-Flop15/2, D Flip-Flop14/2, D Flip-Flop12/2, D Flip-Flop20/2, D Flip-Flop19/2, D Flip-Flop11/2, D Flip-Flop10/2, D Flip-Flop9/2, D Flip-Flop8/2, D Flip-Flop7/2, D Flip-Flop6/2  "clk"
  D Flip-Flop8/1 -> Mux5/4, D Flip-Flop9/1
  D Flip-Flop15/1 -> Mux3/5, D Flip-Flop16/1
  D Flip-Flop16/1 -> Mux3/6, D Flip-Flop17/1
  D Flip-Flop18/1 -> Mux3/8
  D Flip-Flop19/1 -> Mux5/8, D Flip-Flop20/1
  D Flip-Flop11/1 -> Mux5/7, D Flip-Flop19/1
  D Flip-Flop20/1 -> D Flip-Flop12/1, Mux3/1
  conv2/1 -> D Flip-Flop6/1, Mux5/1  "D_in"
  Mux5/1 -> Mux6/1
  Mux3/1 -> Mux6/2
  D_in/1 -> conv2/1
  Clk/1 -> conv/1
  Counter1/1 -> ClkCtr/1, Compare To Constant/1  "clkCtr"
  Compare To Constant/1 -> ?  "condition"
  conv1/1 -> Logical Operator/1, Counter1/2  "rst_"
  Reset/1 -> conv1/1
  Logical Operator/1 -> D Flip-Flop6/3, D Flip-Flop18/3, D Flip-Flop17/3, D Flip-Flop16/3, D Flip-Flop15/3, D Flip-Flop14/3, D Flip-Flop13/3, D Flip-Flop12/3, D Flip-Flop19/3, D Flip-Flop20/3, D Flip-Flop11/3, D Flip-Flop10/3, D Flip-Flop9/3, D Flip-Flop8/3, D Flip-Flop7/3
  Mux6/1 -> Dout/1

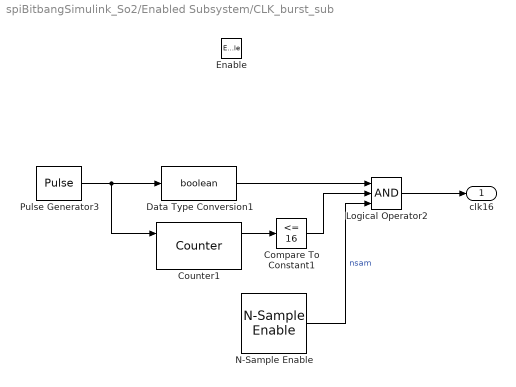
== system spiBitbangSimulink_So2/Enabled Subsystem/CLK_burst_sub ==
  Enable : EnablePort  StatesWhenEnabling=reset
  Compare To Constant1 : simulink/Logic and Bit Operations/Compare To Constant  relop=<=  const=16  OutDataTypeStr=boolean
  Counter1 : dspswit3/Counter  Direction=Down  CountEvent=Rising edge  CounterSize=User defined  MaxCount=16  InitialCount=0  Output=Count and Hit  HitValue=4  ResetInput=on  SamplesPerFrame=1  Ts=1  CntDtype=double  HitDtype=Logical
  Data Type Conversion1 : DataTypeConversion  OutDataTypeStr=boolean
  Logical Operator2 : Logic  Inputs=3  AllPortsSameDT=off  OutDataTypeStr=boolean
  N-Sample Enable : dspswit3/N-Sample Enable  N=16*periSam  ActiveLevel=Low (0)  reset=on  TriggerType=Falling edge  Ts=-1  DataType=Logical
  Pulse Generator3 : DiscretePulseGenerator  Period=periSam  PulseWidth=periSam/2  SampleTime=-1
  clk16 : Outport
  wires:
  Pulse Generator3/1 -> Counter1/1, Data Type Conversion1/1
  Data Type Conversion1/1 -> Logical Operator2/1
  Counter1/1 -> Compare To Constant1/1
  Compare To Constant1/1 -> Logical Operator2/2
  Logical Operator2/1 -> clk16/1
  N-Sample Enable/1 -> Logical Operator2/3  "nsam"

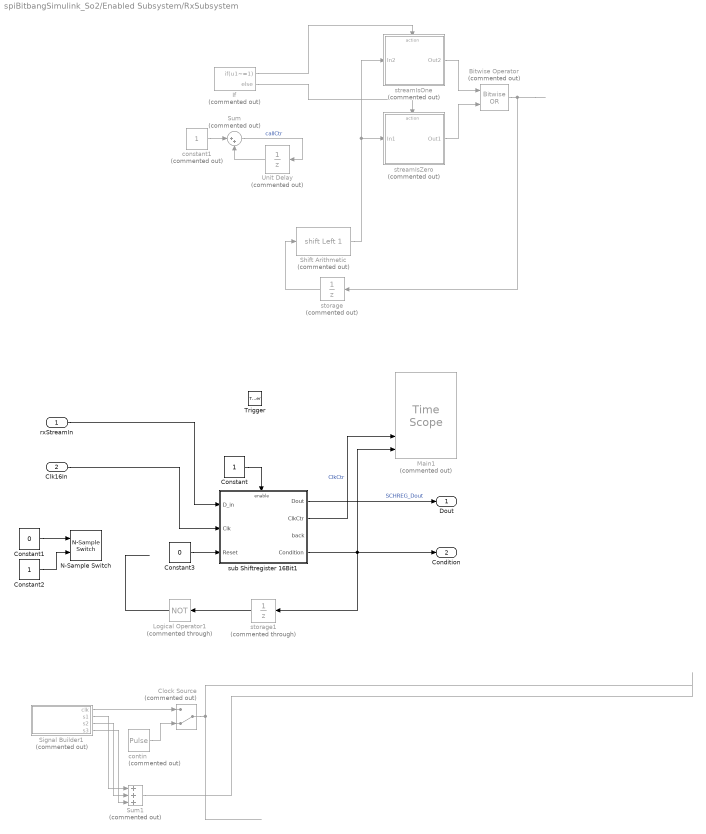
== system spiBitbangSimulink_So2/Enabled Subsystem/RxSubsystem ==
  rxStreamIn : Inport
  Clk16In : Inport  Port=2
  Trigger : TriggerPort
  Bitwise Operator : simulink/Logic and Bit Operations/Bitwise Operator  Commented=on  logicop=OR  UseBitMask=off  NumInputPorts=2  BitMask=bin2dec('11011001')  BitMaskRealWorld=Stored Integer
  Clock Source : ManualSwitch  Commented=on  CurrentSetting=0
  Constant : Constant
  Constant1 : Constant  Value=0  SampleTime=-1
  Constant2 : Constant  SampleTime=-1
  Constant3 : Constant  Value=0  SampleTime=-1
  If : If  Commented=on  IfExpression=u1~=1
  Logical Operator1 : Logic  Commented=through  Operator=NOT  IconShape=distinctive  AllPortsSameDT=off  OutDataTypeStr=boolean
  Main1 : TimeScope  Commented=on  NumInputPorts=6  DefaultConfigurationName=spbscopes.TimeScopeBlockCfg
      settings: CopyFcn=scopeextensions.ScopeBlock.onCoreBlockCopy(gcbh);  DeleteFcn=scopeextensions.ScopeBlock.callback(gcbh, 'onBlockDelete');  PreSaveFcn=scopeextensions.ScopeBlock.callback(gcbh, 'onModelSave');  NameChangeFcn=scopeextensions.ScopeBlock.callback(gcbh, 'onBlockRename');  DestroyFcn=scopeextensions.ScopeBlock.onBlockDestroy(gcbh)  CloseFcn=scopeextensions.ScopeBlock.callback(gcbh, 'onBlockClose');  PreDeleteFcn=scopeextensions.ScopeBlock.callback(gcbh, 'onBlockPreDelete');
  N-Sample Switch : dspswit3/N-Sample Switch  N=30  reset=off  TriggerType=Rising edge  Ts=-1
  Shift Arithmetic : ArithShift  Commented=on  BitShiftNumber=1  BitShiftDirection=Left  DiagnosticForOORShift=Warning  CheckOORBitShift=on
  Signal Builder1 : Subsystem  Tag=STV Subsys  Commented=on  LoadFcn=sigbuilder_block('load');  StartFcn=sigbuilder_block('start');  StopFcn=sigbuilder_block('stop');  ClipboardFcn=sigbuilder_block('clipboard');  TreatAsAtomicUnit=on  mask(Sigbuilder block){}
      mask help: Simulink:masks:SigbuilderBlock_MD
      mask init:
      | if ~strcmp(get_param(bdroot(gcbh),'SimulationStatus'),'stopped') tuvar = sigbuilder_block('maskInit'); end
      settings: CopyFcn=sigbuilder_block('copy');  DeleteFcn=sigbuilder_block('delete');  ModelCloseFcn=sigbuilder_block('modelClose');  PreSaveFcn=sigbuilder_block('preSave');  PauseFcn=sigbuilder_block('pause');  ContinueFcn=sigbuilder_block('continue');  NameChangeFcn=sigbuilder_block('namechange');  OpenFcn=sigbuilder_block('open',[367.5 149.25 803.25 388.5 ]);  CloseFcn=sigbuilder_block('close');
      mask Display: plot(0, 0, 100, 100,[2, 2, 32, 32, 2], [68, 8, 8, 68, 68],[32, 2], [38, 38], [32, 19, 2],[53, 60, 44], [32, 17, 17, 2],[16, 16, 31, 31]);txt = getActiveGroup(gcbh);text(2, 100, txt,'verticalAlignment', 'top');
  Sum : Sum  Commented=on  Inputs=|++  SaturateOnIntegerOverflow=on  InputSameDT=on  OutDataTypeStr=Inherit: Same as first input
  Sum1 : Sum  Commented=on  Inputs=+++  SampleTime=sampleTime
  Unit Delay : UnitDelay  Commented=on
  constant1 : Constant  Commented=on  OutDataTypeStr=int8  LockScale=on
  contin : DiscretePulseGenerator  Commented=on  Period=periSam  PulseWidth=periSam*0.5  SampleTime=sampleTime
  storage : UnitDelay  Commented=on  SampleTime=-1
  storage1 : UnitDelay  Commented=through  SampleTime=-1
  streamIsOne : Subsystem  Commented=on  TreatAsAtomicUnit=on
  streamIsZero : Subsystem  Commented=on  TreatAsAtomicUnit=on
  sub Shiftregister 16Bit1 : Subsystem  TreatAsAtomicUnit=on
  Dout : Outport
  Condition : Outport  Port=2
  wires:
  Sum/1 -> Unit Delay/1  "callCtr"
  constant1/1 -> Sum/1
  Unit Delay/1 -> Sum/2
  Shift Arithmetic/1 -> streamIsOne/1(In2), streamIsZero/1(In1)
  storage/1 -> Shift Arithmetic/1
  If/2 -> streamIsZero/Action
  If/1 -> streamIsOne/Action
  streamIsOne/1(Out2) -> Bitwise Operator/1
  streamIsZero/1(Out1) -> Bitwise Operator/2
  Bitwise Operator/1 -> storage/1
  sub Shiftregister 16Bit1/2(ClkCtr) -> Main1/5  "ClkCtr"
  sub Shiftregister 16Bit1/4(Condition) -> storage1/1, Condition/1, Main1/6
  rxStreamIn/1 -> sub Shiftregister 16Bit1/1(D_in)
  Signal Builder1/3(s2) -> Sum1/2
  Signal Builder1/2(s1) -> Sum1/1
  Signal Builder1/4(s3) -> Sum1/3
  Sum1/1 -> ?
  Clock Source/1 -> ?
  Signal Builder1/1(clk) -> Clock Source/1
  contin/1 -> Clock Source/2
  Clk16In/1 -> sub Shiftregister 16Bit1/2(Clk)
  Constant/1 -> sub Shiftregister 16Bit1/Enable
  Constant1/1 -> N-Sample Switch/1
  Constant2/1 -> N-Sample Switch/2
  Logical Operator1/1 -> ?
  sub Shiftregister 16Bit1/1(Dout) -> Dout/1  "SCHREG_Dout"
  storage1/1 -> Logical Operator1/1
  Constant3/1 -> sub Shiftregister 16Bit1/3(Reset)

== system spiBitbangSimulink_So2/RxSub/DoLockClk ==
  IfAction : ActionPort
  Constant : Constant  SampleTime=-1
  "Reset " : Outport
  wires:
  Constant/1 -> "Reset "/1

== system spiBitbangSimulink_So2/RxSub/NoMoreBusy ==
  In Data : Inport
  IfAction : ActionPort
  Constant : Constant  SampleTime=-1
  Store Buffer : DataStoreWrite  DataStoreName=DataBuff  DataStoreElements=DataBuff
  "Lock " : Outport
  wires:
  In Data/1 -> Store Buffer/1
  Constant/1 -> "Lock "/1

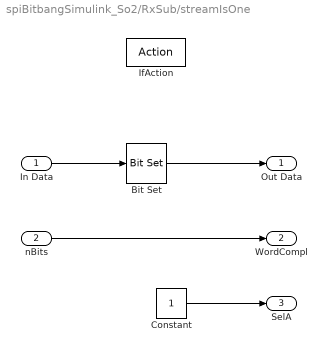
== system spiBitbangSimulink_So2/RxSub/streamIsOne ==
  In Data : Inport
  nBits : Inport  Port=2
  IfAction : ActionPort
  Bit Set : simulink/Logic and Bit Operations/Bit Set  iBit=0
  Constant : Constant  OutDataTypeStr=Inherit: Inherit via back propagation  SampleTime=-1
  Out Data : Outport
  WordCompl : Outport  Port=2
  SelA : Outport  Port=3
  wires:
  In Data/1 -> Bit Set/1
  Bit Set/1 -> Out Data/1
  nBits/1 -> WordCompl/1
  Constant/1 -> SelA/1

== system spiBitbangSimulink_So2/RxSub/streamIsOne1 ==
  nBits : Inport
  IfAction : ActionPort
  WordCompl : Outport  OutDataTypeStr=uint8
  wires:
  nBits/1 -> WordCompl/1

== system spiBitbangSimulink_So2/RxSub/streamIsZero ==
  In Data : Inport
  nBits : Inport  Port=2
  IfAction : ActionPort
  Bit Clear : simulink/Logic and Bit Operations/Bit Clear  iBit=0
  Out Data : Outport
  WordCompl : Outport  Port=2
  wires:
  In Data/1 -> Bit Clear/1
  Bit Clear/1 -> Out Data/1
  nBits/1 -> WordCompl/1

== system spiBitbangSimulink_So2/Triggered Subsystem/streamIsOne ==
  In2 : Inport  OutDataTypeStr=int8
  IfAction : ActionPort  ActionType=then
  Bit Set : simulink/Logic and Bit Operations/Bit Set  iBit=0
  Out2 : Outport  OutDataTypeStr=uint8
  wires:
  In2/1 -> Bit Set/1
  Bit Set/1 -> Out2/1

== system spiBitbangSimulink_So2/Triggered Subsystem/streamIsZero ==
  In1 : Inport  OutDataTypeStr=int8
  IfAction : ActionPort  ActionType=else
  Bit Clear : simulink/Logic and Bit Operations/Bit Clear  iBit=0
  Out1 : Outport  OutDataTypeStr=uint8
  wires:
  In1/1 -> Bit Clear/1
  Bit Clear/1 -> Out1/1

== system spiBitbangSimulink_So2/Enabled Subsystem/RxSubsystem/Signal Builder1 ==
  Demux : Demux  Tag=STV Demux
  FromWs : FromWorkspace  Tag=STV FromWs  VariableName=tuvar  SampleTime=0
      SigBuilderData=|
      | common.afterFinalStr = 'Extrapolate'
      | common.sampleTime = '0'
      | dataSet.timeRange = [0 0.00032]
      | dataSet.name = 'Group 1'
      | sbobj.Groups.Name = 'Group 1'
      | sbobj.Groups.Signals(1).Name = 'clk'
      | sbobj.Groups.Signals(1).XData = [0 1e-05 1e-05 2e-05 2e-05 3e-05 3e-05 4e-05 4e-05 5e-05 5e-05 6e-05 6e-05 7e-05 7e-05 8e-05 8e-05 9e-05 9e-05 0.0001 0.0001 0.00011 0.00011 0.00012 0.00012 0.00013 0.00013 0.00014 0.00014 0.00015 0.00015 0.00016 0.00016 0.00017 0.00017 0.00018 0.00018 0.00019 0.00019 0.0002 0.0002 0.00021 0.00021 0.00022 0.00022 0.00023 0.00023 0.00024 0.00024 0.00025 0.00025 0.00026 0.00026 0.00027 0.00027 0.00028 0.00028 0.00029 0.00029 0.0003 0.0003 0.00031 0.00031 0.00032]
      | sbobj.Groups.Signals(1).YData = [1 1 0 0 1 1 0 0 1 1 0 0 1 1 0 0 1 1 0 0 1 1 0 0 1 1 0 0 1 1 0 0 1 1 0 0 1 1 0 0 1 1 0 0 1 1 0 0 1 1 0 0 1 1 0 0 1 1 0 0 1 1 0 0]
      | sbobj.Groups.Signals(2).Name = 's1'
      | sbobj.Groups.Signals(2).XData = [0 5e-06 5e-06 5.45e-05 5.45e-05 0.00032]
      | sbobj.Groups.Signals(2).YData = [0 0 1 1 0 0]
      | sbobj.Groups.Signals(3).Name = 's2'
      | sbobj.Groups.Signals(3).XData = [0 0.0001475 0.0001475 0.000196 0.000196 0.00032]
      | sbobj.Groups.Signals(3).YData = [0 0 1 1 0 0]
      | sbobj.Groups.Signals(4).Name = 's3'
      | sbobj.Groups.Signals(4).XData = [0 0.000237 0.000237 0.000297 0.000297 0.00032]
      | sbobj.Groups.Signals(4).YData = [0 0 1 1 0 0]
      | sbobj.Groups.TimeRange = [0 0.00032]
  clk : Outport  Tag=STV Outport
  s1 : Outport  Tag=STV Outport  Port=2
  s2 : Outport  Tag=STV Outport  Port=3
  s3 : Outport  Tag=STV Outport  Port=4
  wires:
  FromWs/1 -> Demux/1
  Demux/1 -> clk/1
  Demux/2 -> s1/1
  Demux/3 -> s2/1
  Demux/4 -> s3/1

== system spiBitbangSimulink_So2/Enabled Subsystem/RxSubsystem/streamIsOne ==
  In2 : Inport  OutDataTypeStr=int8
  IfAction : ActionPort  ActionType=then
  Bit Set : simulink/Logic and Bit Operations/Bit Set  iBit=0
  Out2 : Outport  OutDataTypeStr=uint8
  wires:
  In2/1 -> Bit Set/1
  Bit Set/1 -> Out2/1

== system spiBitbangSimulink_So2/Enabled Subsystem/RxSubsystem/streamIsZero ==
  In1 : Inport  OutDataTypeStr=int8
  IfAction : ActionPort  ActionType=else
  Bit Clear : simulink/Logic and Bit Operations/Bit Clear  iBit=0
  Out1 : Outport  OutDataTypeStr=uint8
  wires:
  In1/1 -> Bit Clear/1
  Bit Clear/1 -> Out1/1

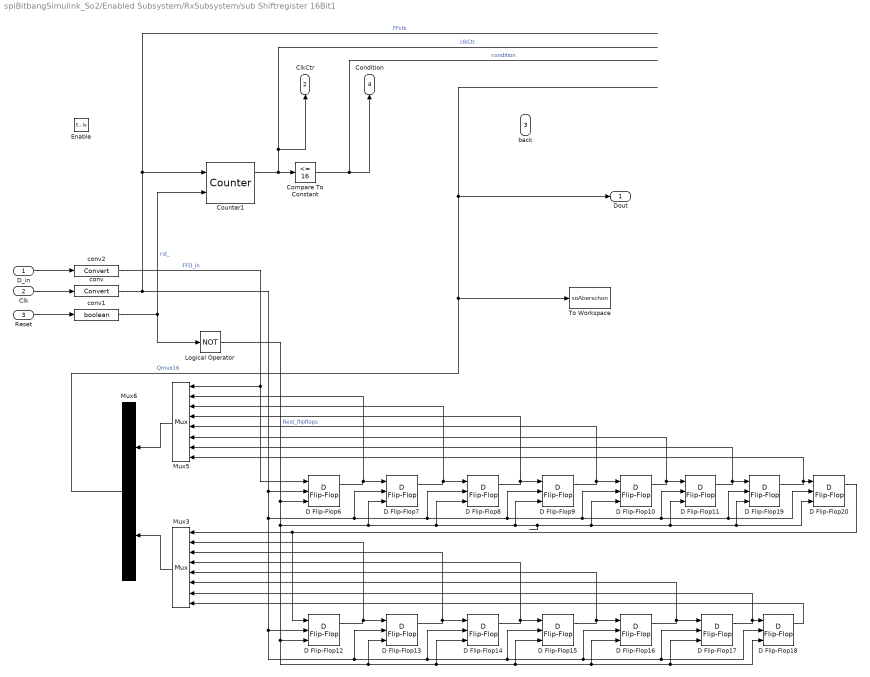
== system spiBitbangSimulink_So2/Enabled Subsystem/RxSubsystem/sub Shiftregister 16Bit1 ==
  D_in : Inport
  Clk : Inport  Port=2
  Reset : Inport  Port=3
  Enable : EnablePort  StatesWhenEnabling=reset
  Compare To Constant : simulink/Logic and Bit Operations/Compare To Constant  relop=<=  const=16  OutDataTypeStr=boolean  ZeroCross=off
  Counter1 : dspswit3/Counter  Direction=Up  CountEvent=Rising edge  CounterSize=User defined  MaxCount=255  InitialCount=0  Output=Count and Hit  HitValue=32  ResetInput=on  SamplesPerFrame=1  Ts=1  CntDtype=double  HitDtype=Boolean
  D Flip-Flop{6..20} (15 alike) : simulink_extras/Flip Flops/D Flip-Flop
  Logical Operator : Logic  Operator=NOT  IconShape=distinctive  AllPortsSameDT=off  OutDataTypeStr=boolean
  Mux3 : Mux  Inputs=8
  Mux5 : Mux  Inputs=8
  Mux6 : Mux  Inputs=2
  To Workspace : ToWorkspace  VariableName=soAberschon  SampleTime=-1  SaveFormat=Timeseries
  conv : DataTypeConversion  LockScale=on
  conv1 : DataTypeConversion  OutDataTypeStr=boolean
  conv2 : DataTypeConversion
  Dout : Outport
  ClkCtr : Outport  Port=2
  back : Outport  Port=3
  Condition : Outport  Port=4
  wires:
  D Flip-Flop6/1 -> Mux5/2, D Flip-Flop7/1
  D Flip-Flop7/1 -> Mux5/3, D Flip-Flop8/1
  D Flip-Flop9/1 -> Mux5/5, D Flip-Flop10/1
  D Flip-Flop10/1 -> Mux5/6, D Flip-Flop11/1
  D Flip-Flop12/1 -> Mux3/2, D Flip-Flop13/1
  D Flip-Flop13/1 -> Mux3/3, D Flip-Flop14/1
  D Flip-Flop14/1 -> Mux3/4, D Flip-Flop15/1
  D Flip-Flop17/1 -> Mux3/7, D Flip-Flop18/1
  conv/1 -> D Flip-Flop13/2, D Flip-Flop16/2, D Flip-Flop17/2, D Flip-Flop18/2, D Flip-Flop15/2, D Flip-Flop14/2, D Flip-Flop12/2, D Flip-Flop20/2, D Flip-Flop19/2, D Flip-Flop11/2, D Flip-Flop10/2, D Flip-Flop9/2, D Flip-Flop8/2, D Flip-Flop7/2, D Flip-Flop6/2, Counter1/1  "FFclk"
  D Flip-Flop8/1 -> Mux5/4, D Flip-Flop9/1
  D Flip-Flop15/1 -> Mux3/5, D Flip-Flop16/1
  D Flip-Flop16/1 -> Mux3/6, D Flip-Flop17/1
  D Flip-Flop18/1 -> Mux3/8
  D Flip-Flop19/1 -> Mux5/8, D Flip-Flop20/1
  D Flip-Flop11/1 -> Mux5/7, D Flip-Flop19/1
  D Flip-Flop20/1 -> D Flip-Flop12/1, Mux3/1
  conv2/1 -> D Flip-Flop6/1, Mux5/1  "FFD_in"
  Mux5/1 -> Mux6/1
  Mux3/1 -> Mux6/2
  D_in/1 -> conv2/1
  Clk/1 -> conv/1
  Counter1/1 -> ClkCtr/1, Compare To Constant/1  "clkCtr"
  Compare To Constant/1 -> Condition/1  "condition"
  conv1/1 -> Logical Operator/1, Counter1/2  "rst_"
  Reset/1 -> conv1/1
  Logical Operator/1 -> D Flip-Flop6/3, D Flip-Flop18/3, D Flip-Flop17/3, D Flip-Flop16/3, D Flip-Flop15/3, D Flip-Flop14/3, D Flip-Flop13/3, D Flip-Flop12/3, D Flip-Flop19/3, D Flip-Flop20/3, D Flip-Flop11/3, D Flip-Flop10/3, D Flip-Flop9/3, D Flip-Flop8/3, D Flip-Flop7/3  "Rest_flipflops"
  Mux6/1 -> To Workspace/1, Dout/1  "Qmux16"

== stateflow chart spiBitbangSimulink_So2/Chart ==
  state on
  state off
  on -> off : switch/lightSwitch=0;
  off -> on : switch/lightSwitch=1;
  (default) -> off : /lightSwitch=0;
  data: lightSwitch output double
  events: switch input EITHER_EDGE_EVENT
